simulink model "interp_test"  (R2018a)
settings: Solver=VariableStepAuto  StartTime=0.0  StopTime=10.0  RelTol=1e-3
undefined symbols (not defined in the file): a, a1, a_10t, a_space, atable, table_2D10, table_2D20, table_3D, table_3Dfor_mass, u_space, utableall, v, V, v_space, V_table, vtable
settings Model: Creator=cidi-xh  LastModifiedBy=cidi-xh

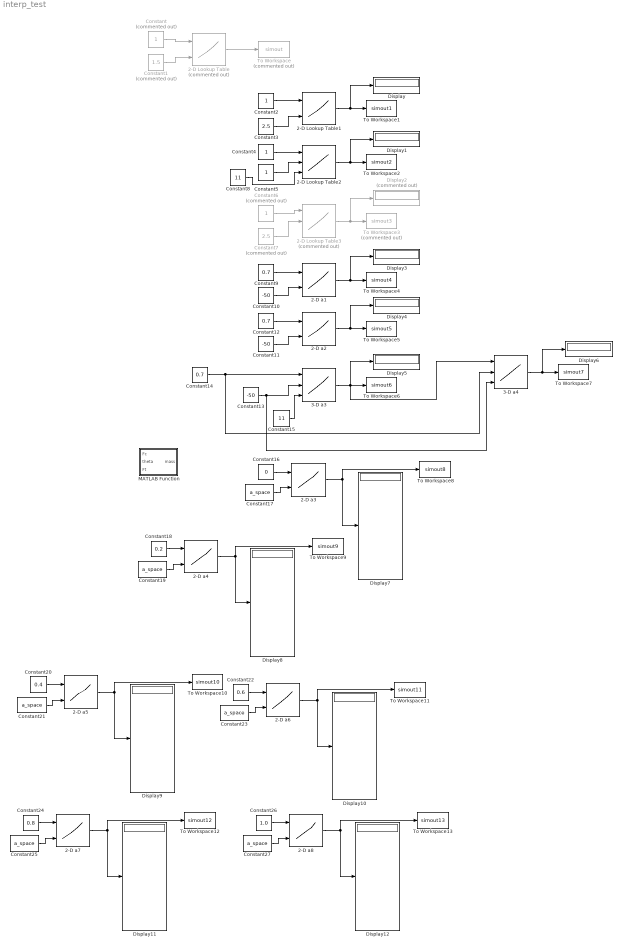
== system interp_test ==
  2-D Lookup Table : Lookup_n-D  Commented=on  BreakpointsForDimension1=v  BreakpointsForDimension2=a  Table=V  InternalRulePriority=Speed  RndMeth=Simplest  InputSameDT=on
  2-D Lookup Table1 : Lookup_n-D  BreakpointsForDimension1=[1:3]  BreakpointsForDimension2=[1:3]  InternalRulePriority=Speed  RndMeth=Simplest  InputSameDT=on
  2-D Lookup Table2 : Lookup_n-D  NumberOfTableDimensions=3  BreakpointsForDimension1=[-60 -50]  BreakpointsForDimension2="[0 0.6  0.8 1]"  BreakpointsForDimension3=[10 20]  Table=a1  InternalRulePriority=Speed  RndMeth=Simplest  InputSameDT=on
  2-D Lookup Table3 : Lookup_n-D  Commented=on  NumberOfTableDimensions=3  BreakpointsForDimension1=a_10t  BreakpointsForDimension2=[0 1]  BreakpointsForDimension3=[-60 -50]  Table=V_table  InternalRulePriority=Speed  RndMeth=Simplest  InputSameDT=on
  2-D a1 : Lookup_n-D  BreakpointsForDimension1=v(1:6,1)  BreakpointsForDimension2=[-60 -50]  BreakpointsForDimension3=[-60 -50]  Table=table_2D10  InternalRulePriority=Speed  RndMeth=Simplest  InputSameDT=on
  2-D a2 : Lookup_n-D  BreakpointsForDimension1=v(1:6,1)  BreakpointsForDimension2=[-60 -50]  BreakpointsForDimension3=[-60 -50]  Table=table_2D20  InternalRulePriority=Speed  RndMeth=Simplest  InputSameDT=on
  2-D a{3..8} (6 alike) : Lookup_n-D  BreakpointsForDimension1=vtable  BreakpointsForDimension2=atable  BreakpointsForDimension3=[-60 -50]  Table=utableall  InternalRulePriority=Speed  RndMeth=Simplest  InputSameDT=on
  3-D a3 : Lookup_n-D  NumberOfTableDimensions=3  BreakpointsForDimension1=v(1:6,1)  BreakpointsForDimension2=[-60 -50]  BreakpointsForDimension3=[10 20]  Table=table_3D  InternalRulePriority=Speed  RndMeth=Simplest  InputSameDT=on
  3-D a4 : Lookup_n-D  NumberOfTableDimensions=3  BreakpointsForDimension1=a_space  BreakpointsForDimension2=v_space  BreakpointsForDimension3=u_space  Table=table_3Dfor_mass  InternalRulePriority=Speed  RndMeth=Simplest  InputSameDT=on
  Constant : Constant  Commented=on
  Constant1 : Constant  Commented=on  Value=1.5
  Constant10 : Constant  Value=-50
  Constant11 : Constant  Value=-50
  Constant12 : Constant  Value=0.7
  Constant13 : Constant  Value=-50
  Constant14 : Constant  Value=0.7
  Constant15 : Constant  Value=11
  Constant16 : Constant  Value=0
  Constant{17,19,21,23,25,27} (6 alike) : Constant  Value=a_space
  Constant18 : Constant  Value=0.2
  Constant2 : Constant
  Constant20 : Constant  Value=0.4
  Constant22 : Constant  Value=0.6
  Constant24 : Constant  Value=0.8
  Constant26 : Constant  Value=1.0
  Constant3 : Constant  Value=2.5
  Constant4 : Constant
  Constant5 : Constant
  Constant6 : Constant  Commented=on
  Constant7 : Constant  Commented=on  Value=2.5
  Constant8 : Constant  Value=11
  Constant9 : Constant  Value=0.7
  Display{,1,3..12} (12 alike) : Display
  Display2 : Display  Commented=on
  MATLAB Function : MATLAB Function  TreatAsAtomicUnit=on
  To Workspace : ToWorkspace  Commented=on  VariableName=simout  SaveFormat=Timeseries  SampleTime=-1
  To Workspace1 : ToWorkspace  VariableName=simout1  SaveFormat=Timeseries  SampleTime=-1
  To Workspace10 : ToWorkspace  VariableName=simout10  SampleTime=-1
  To Workspace11 : ToWorkspace  VariableName=simout11  SampleTime=-1
  To Workspace12 : ToWorkspace  VariableName=simout12  SampleTime=-1
  To Workspace13 : ToWorkspace  VariableName=simout13  SampleTime=-1
  To Workspace2 : ToWorkspace  VariableName=simout2  SaveFormat=Timeseries  SampleTime=-1
  To Workspace3 : ToWorkspace  Commented=on  VariableName=simout3  SaveFormat=Timeseries  SampleTime=-1
  To Workspace4 : ToWorkspace  VariableName=simout4  SaveFormat=Timeseries  SampleTime=-1
  To Workspace5 : ToWorkspace  VariableName=simout5  SaveFormat=Timeseries  SampleTime=-1
  To Workspace6 : ToWorkspace  VariableName=simout6  SaveFormat=Timeseries  SampleTime=-1
  To Workspace7 : ToWorkspace  VariableName=simout7  SaveFormat=Timeseries  SampleTime=-1
  To Workspace8 : ToWorkspace  VariableName=simout8  SampleTime=-1
  To Workspace9 : ToWorkspace  VariableName=simout9  SampleTime=-1
  wires:
  Constant/1 -> 2-D Lookup Table/1
  Constant1/1 -> 2-D Lookup Table/2
  2-D Lookup Table/1 -> To Workspace/1
  Constant2/1 -> 2-D Lookup Table1/1
  Constant3/1 -> 2-D Lookup Table1/2
  2-D Lookup Table1/1 -> Display/1, To Workspace1/1
  2-D Lookup Table2/1 -> To Workspace2/1, Display1/1
  Constant5/1 -> 2-D Lookup Table2/2
  Constant4/1 -> 2-D Lookup Table2/1
  Constant6/1 -> 2-D Lookup Table3/1
  Constant7/1 -> 2-D Lookup Table3/2
  2-D Lookup Table3/1 -> Display2/1, To Workspace3/1
  Constant8/1 -> 2-D Lookup Table2/3
  2-D a1/1 -> To Workspace4/1, Display3/1
  Constant10/1 -> 2-D a1/2
  Constant9/1 -> 2-D a1/1
  Constant12/1 -> 2-D a2/1
  Constant11/1 -> 2-D a2/2
  2-D a2/1 -> Display4/1, To Workspace5/1
  Constant13/1 -> 3-D a3/2, 3-D a4/3
  Constant15/1 -> 3-D a3/3
  3-D a3/1 -> 3-D a4/1, To Workspace6/1, Display5/1
  Constant14/1 -> 3-D a3/1, 3-D a4/2
  3-D a4/1 -> Display6/1, To Workspace7/1
  Constant16/1 -> 2-D a3/1
  Constant17/1 -> 2-D a3/2
  2-D a3/1 -> Display7/1, To Workspace8/1
  2-D a4/1 -> To Workspace9/1, Display8/1
  Constant19/1 -> 2-D a4/2
  Constant18/1 -> 2-D a4/1
  Constant20/1 -> 2-D a5/1
  Constant21/1 -> 2-D a5/2
  2-D a5/1 -> Display9/1, To Workspace10/1
  2-D a6/1 -> To Workspace11/1, Display10/1
  Constant23/1 -> 2-D a6/2
  Constant22/1 -> 2-D a6/1
  Constant24/1 -> 2-D a7/1
  Constant25/1 -> 2-D a7/2
  2-D a7/1 -> Display11/1, To Workspace12/1
  2-D a8/1 -> To Workspace13/1, Display12/1
  Constant27/1 -> 2-D a8/2
  Constant26/1 -> 2-D a8/1

== matlab function interp_test/MATLAB Function ==
  data: mass output; Fc input; theta input; Ft input
function mass = fcn(Fc,theta,Ft)
na = 1;nb = 1;d = 3; %structure parameters
uk = 0;%initial value of system input
yk = 0;%initial value of system output
L = 1;
g = 9.8;%unit:m/s^2
%theta = 0;% slope of the road,unit:degree or rad?

xi = sqrt(0.1) * randn(L,1);%white noise 
i = -sin(theta);
phi = g * i;

Fg = Fc - Ft - xi;
mass = 10000;% initial value of the object to be estimated
% persistent mass_last;
% mass_last 
P = 10^6 * eye(na - 1 + nb - 1 + 1);
% Fg = phi * m + xi; % y(k) = phi(k)' * theta + xi 标准的二乘递归形式
% mass_data 

% RLS algorithm
K = P * phi / (1 + phi' * P * phi);
% mass = mass_last + K * (Fg - phi' * mass_last);
mass = mass + K * (Fg - phi' * mass);
P = (eye(na - 1 + nb - 1 + 1) - K * phi') * P;

% mass_last = mass;
